simulink model "simulink_tuan1"  (R2019a)
settings: Solver=VariableStepAuto  StartTime=0.0  StopTime=10  RelTol=1e-3
libraries: simulink x1
settings Model: Creator=inhuo  LastModifiedBy=inhuo

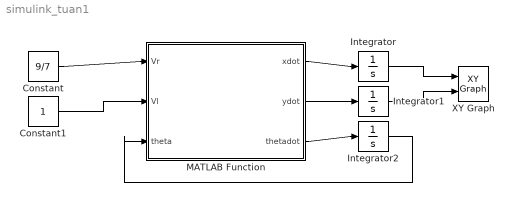
== system simulink_tuan1 ==
  Constant : Constant  Value=9/7
  Constant1 : Constant
  Integrator : Integrator
  Integrator1 : Integrator
  Integrator2 : Integrator
  MATLAB Function : MATLAB Function  TreatAsAtomicUnit=on
  XY Graph : simulink/Sinks/XY Graph  xmin=-4  xmax=4  ymin=0  ymax=5  st=-1
  wires:
  Constant/1 -> MATLAB Function/1(Vr)
  Constant1/1 -> MATLAB Function/2(Vl)
  MATLAB Function/1(xdot) -> Integrator/1
  MATLAB Function/2(ydot) -> Integrator1/1
  MATLAB Function/3(thetadot) -> Integrator2/1
  Integrator2/1 -> MATLAB Function/3(theta)
  Integrator/1 -> XY Graph/1
  Integrator1/1 -> XY Graph/2

== matlab function simulink_tuan1/MATLAB Function ==
  data: Vr input; xdot output; Vl input; theta input; ydot output; thetadot output
function [xdot, ydot, thetadot] = fcn(Vr, Vl, theta)

d=0.5; % axial space
xdot = (Vr + Vl)/2 *cos(theta);
ydot = (Vr + Vl)/2 *sin(theta);
thetadot = (Vr - Vl)/d;
